simulink model "Assignment_M1_simulink"  (R2019b)
settings: Solver=VariableStepAuto  StartTime=0.0  StopTime=0.1  RelTol=1e-3
values from neighbouring files (symbols this model uses):
  A = [0 0 0 1 0 ... (first row only)    [Assignment_M1.m]    (also in M2_David.m)
  B = [0 0 0 K_T/(R*J_1) 0 ... (first row only)    [Assignment_M1.m]    (also in M2_David.m = [0 0; 0 0; 0 1/b; Kt/(R*J1) 0; 0 0])
  C_1 = [0 1 0 0 0 ... (first row only)    [Assignment_M1.m]
  C_2 = [0 0 0 -K_E/R 0 ... (first row only)    [Assignment_M1.m]
  D_1 = 20    [Assignment_M1.m]
  D_2 = 2    [Assignment_M1.m]
settings Model: Creator=albin  LastModifiedBy=albin

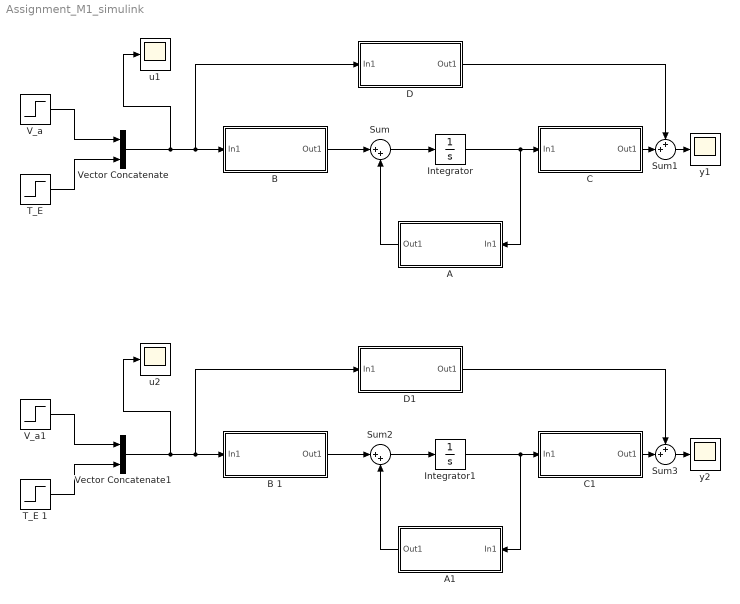
== system Assignment_M1_simulink ==
  A : Subsystem
  A1 : Subsystem
  "B " : Subsystem
  B 1 : Subsystem
  C : Subsystem
  C1 : Subsystem
  D : Subsystem
  D1 : Subsystem
  Integrator : Integrator
  Integrator1 : Integrator
  Sum : Sum  Inputs=|++
  Sum1 : Sum  Inputs=++|
  Sum2 : Sum  Inputs=|++
  Sum3 : Sum  Inputs=++|
  "T_E " : Step  Time=5/100  After=-0.1  SampleTime=0
  T_E 1 : Step  Time=5/100  After=-0.1  SampleTime=0
  V_a : Step  Time=2/100  After=10  SampleTime=0
  V_a1 : Step  Time=2/100  After=10  SampleTime=0
  Vector Concatenate : Concatenate
  Vector Concatenate1 : Concatenate
  "u1 " : Scope
  "u2 " : Scope
  "y1 " : Scope
  "y2 " : Scope
  wires:
  Sum/1 -> Integrator/1
  Integrator/1 -> A/1(In1), C/1(In1)
  A/1(Out1) -> Sum/2
  "B "/1(Out1) -> Sum/1
  V_a/1 -> Vector Concatenate/1
  "T_E "/1 -> Vector Concatenate/2
  Vector Concatenate/1 -> "u1 "/1, D/1(In1), "B "/1(In1)
  D/1(Out1) -> Sum1/1
  C/1(Out1) -> Sum1/2
  Sum1/1 -> "y1 "/1
  Sum3/1 -> "y2 "/1
  C1/1(Out1) -> Sum3/2
  Sum2/1 -> Integrator1/1
  B 1/1(Out1) -> Sum2/1
  Integrator1/1 -> A1/1(In1), C1/1(In1)
  V_a1/1 -> Vector Concatenate1/1
  A1/1(Out1) -> Sum2/2
  Vector Concatenate1/1 -> "u2 "/1, D1/1(In1), B 1/1(In1)
  D1/1(Out1) -> Sum3/1
  T_E 1/1 -> Vector Concatenate1/2

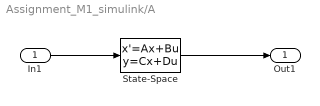
== system Assignment_M1_simulink/A ==
  In1 : Inport
  State-Space : StateSpace  A=[]  B=[]  C=[]  D=A  InitialCondition=0
  Out1 : Outport
  wires:
  In1/1 -> State-Space/1
  State-Space/1 -> Out1/1

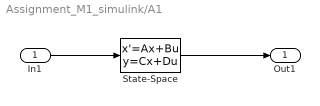
== system Assignment_M1_simulink/A1 ==
  In1 : Inport
  State-Space : StateSpace  A=[]  B=[]  C=[]  D=A  InitialCondition=0
  Out1 : Outport
  wires:
  In1/1 -> State-Space/1
  State-Space/1 -> Out1/1

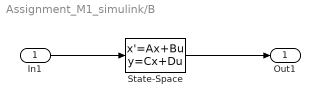
== system Assignment_M1_simulink/B  ==
  In1 : Inport
  State-Space : StateSpace  A=[]  B=[]  C=[]  D=B  InitialCondition=0
  Out1 : Outport
  wires:
  In1/1 -> State-Space/1
  State-Space/1 -> Out1/1

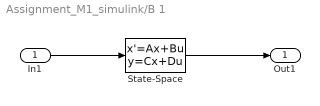
== system Assignment_M1_simulink/B 1 ==
  In1 : Inport
  State-Space : StateSpace  A=[]  B=[]  C=[]  D=B  InitialCondition=0
  Out1 : Outport
  wires:
  In1/1 -> State-Space/1
  State-Space/1 -> Out1/1

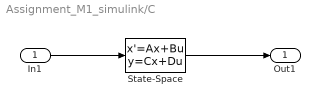
== system Assignment_M1_simulink/C ==
  In1 : Inport
  State-Space : StateSpace  A=[]  B=[]  C=[]  D=C_1  InitialCondition=0
  Out1 : Outport
  wires:
  In1/1 -> State-Space/1
  State-Space/1 -> Out1/1

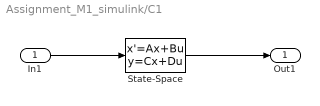
== system Assignment_M1_simulink/C1 ==
  In1 : Inport
  State-Space : StateSpace  A=[]  B=[]  C=[]  D=C_2  InitialCondition=0
  Out1 : Outport
  wires:
  In1/1 -> State-Space/1
  State-Space/1 -> Out1/1

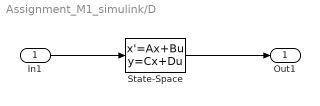
== system Assignment_M1_simulink/D ==
  In1 : Inport
  State-Space : StateSpace  A=[]  B=[]  C=[]  D=D_1  InitialCondition=0
  Out1 : Outport
  wires:
  In1/1 -> State-Space/1
  State-Space/1 -> Out1/1

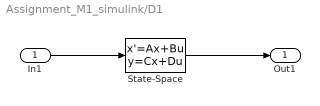
== system Assignment_M1_simulink/D1 ==
  In1 : Inport
  State-Space : StateSpace  A=[]  B=[]  C=[]  D=D_2  InitialCondition=0
  Out1 : Outport
  wires:
  In1/1 -> State-Space/1
  State-Space/1 -> Out1/1
